simulink model "TrafficLights"  (R2017b)
settings: Solver=FixedStepDiscrete  StartTime=0.0  StopTime=10.0  RelTol=1e-3
settings Model: Creator=engdo  LastModifiedBy=engdo
settings OptimizationCC: DefaultParameterBehavior=Inlined  PassReuseOutputArgsAs=Individual arguments
settings DebuggingCC: ParameterTunabilityLossMsg=error
settings SFSimCC: MATLABDynamicMemAlloc=off
settings RTWCC: SystemTargetFile=ert.tlc  GenCodeOnly=on  TemplateMakefile=ert_default_tmf  GenerateReport=on  IncludeHyperlinkInReport=on  LaunchReport=on  GenerateTraceInfo=on  GenerateTraceReport=on  GenerateTraceReportSl=on  GenerateTraceReportSf=on  GenerateTraceReportEml=on  GenerateWebview=on
settings CodeAppCC: ForceParamTrailComments=on  IgnoreCustomStorageClasses=off  OperatorAnnotations=on  SimulinkDataObjDesc=on  SFDataObjDesc=on  InsertBlockDesc=on
settings ERTTargetCC: TargetLangStandard=C99 (ISO)  GenerateSampleERTMain=on  InlinedParameterPlacement=NonHierarchical  ERTCustomFileTemplate=example_file_process.tlc  EnableUserReplacementTypes=on

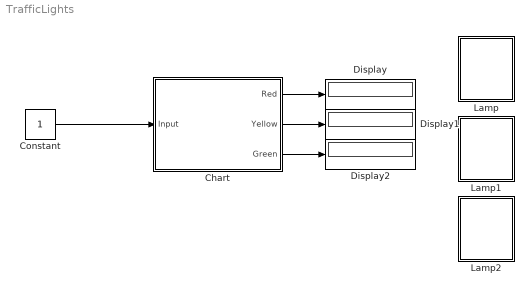
== system TrafficLights ==
  Chart : Stateflow chart  TreatAsAtomicUnit=on
  Constant : Constant
  Display : Display
  Display1 : Display
  Display2 : Display
  Lamp : Subsystem  DialogController=hmiCreateDDGDialog  IsWebBlock=on  mask(MWDashboardBlock){webBlockId=e1e85512-e892-4198-a3b8-63d555df0705, webBlockType=lamp, ShowInLibBrowser=on, ShowInitialText=on, HMISrcModelName=StateFloww}
      mask prompts: webBlockType "WebBlock Type"; HMISrcModelName "Source Model"
      mask help: SimulinkHMI:dialogs:LampDialogDesc
      mask Help: helpview([docroot '/mapfiles/simulink.map'], 'hmi_lamp')
      mask Display:
      | if strcmp(get_param(bdroot(gcb),'BlockDiagramType'), 'library')
      |     image([(matlabroot) '/toolbox/simulink/hmi/icons/Lamp.png']);
      | end
  Lamp1 : Subsystem  DialogController=hmiCreateDDGDialog  IsWebBlock=on  mask(MWDashboardBlock){webBlockId=e9963900-ed50-46ad-a029-e7c8b6dd37e6, webBlockType=lamp, ShowInLibBrowser=on, ShowInitialText=on, HMISrcModelName=StateFloww}
      mask prompts: webBlockType "WebBlock Type"; HMISrcModelName "Source Model"
      mask help: SimulinkHMI:dialogs:LampDialogDesc
      mask Help: helpview([docroot '/mapfiles/simulink.map'], 'hmi_lamp')
      mask Display:
      | if strcmp(get_param(bdroot(gcb),'BlockDiagramType'), 'library')
      |     image([(matlabroot) '/toolbox/simulink/hmi/icons/Lamp.png']);
      | end
  Lamp2 : Subsystem  DialogController=hmiCreateDDGDialog  IsWebBlock=on  mask(MWDashboardBlock){webBlockId=dd39d1b8-d3c7-482b-b3f9-03e9355c6053, webBlockType=lamp, ShowInLibBrowser=on, ShowInitialText=on, HMISrcModelName=StateFloww}
      mask prompts: webBlockType "WebBlock Type"; HMISrcModelName "Source Model"
      mask help: SimulinkHMI:dialogs:LampDialogDesc
      mask Help: helpview([docroot '/mapfiles/simulink.map'], 'hmi_lamp')
      mask Display:
      | if strcmp(get_param(bdroot(gcb),'BlockDiagramType'), 'library')
      |     image([(matlabroot) '/toolbox/simulink/hmi/icons/Lamp.png']);
      | end
  wires:
  Constant/1 -> Chart/1(Input)
  Chart/3(Green) -> Display2/1
  Chart/2(Yellow) -> Display1/1
  Chart/1(Red) -> Display/1

== system TrafficLights/Lamp ==

== system TrafficLights/Lamp1 ==

== system TrafficLights/Lamp2 ==

== stateflow chart TrafficLights/Chart ==
  state ON
  state TrafficLights
  state OFF
  state RedLight
    entry:
    Red=1;
    Yellow=0;
    Green=0;
    exit:
    Red=0;
    Yellow=0;
    Green=0;
  state YellowLight
    entry:
    Red=0;
    Yellow=1;
    Green=0;
    exit:
    Red=0;
    Yellow=0;
    Green=0;
  state GreenLight
    entry:
    Red=0;
    Yellow=0;
    Green=1;
    exit:
    Red=0;
    Yellow=0;
    Green=0;
  (default) -> TrafficLights
  TrafficLights -> ON [order 1] : [Input==1]
  TrafficLights -> OFF [order 2] : [Input==0]
  ON -> RedLight
  GreenLight -> RedLight : after(300, sec)
  RedLight -> YellowLight : after(300, sec)
  YellowLight -> GreenLight : after(300, sec)
  data: Input input; Red output; Yellow output; Green output
